simulink model "MT23PED006_SVPWM_OVERMODULATION_SUBHA_DAS"  (R2023b)
settings: Solver=ode23t  StartTime=0.0  StopTime=0.1  MaxStep=1e-6  RelTol=1e-3
model workspace (MAT data in the model file):
  Fs = 2400
  Ma = 0.66
  Ts = 0.000416666666667
  Vdc = 560
  f = 50
libraries: spsVoltageMeasurementLib x6, spsIGBTDiodeLib x6, spsSeriesRLCBranchLib x5, spsGroundLib x2, spsDCVoltageSourceLib x1, dspstat3 x1, spsThreePhaseVIMeasurementLib x1, mcbutilslib x1, sps_lib x1
settings Model: Creator=ixale  LastModifiedBy=ixale
settings DataIOCC: ReturnWorkspaceOutputs=off

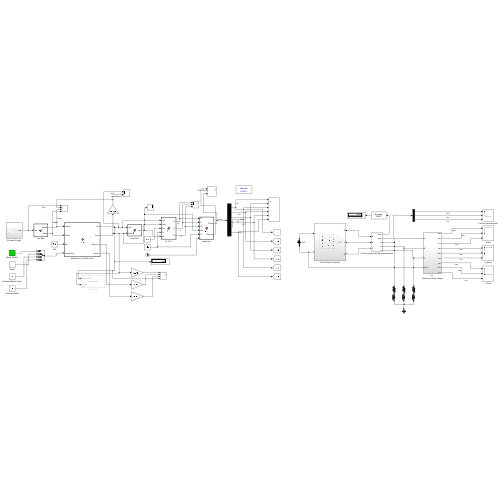
[thumbnail: Simulink's stored preview of the top-level diagram]
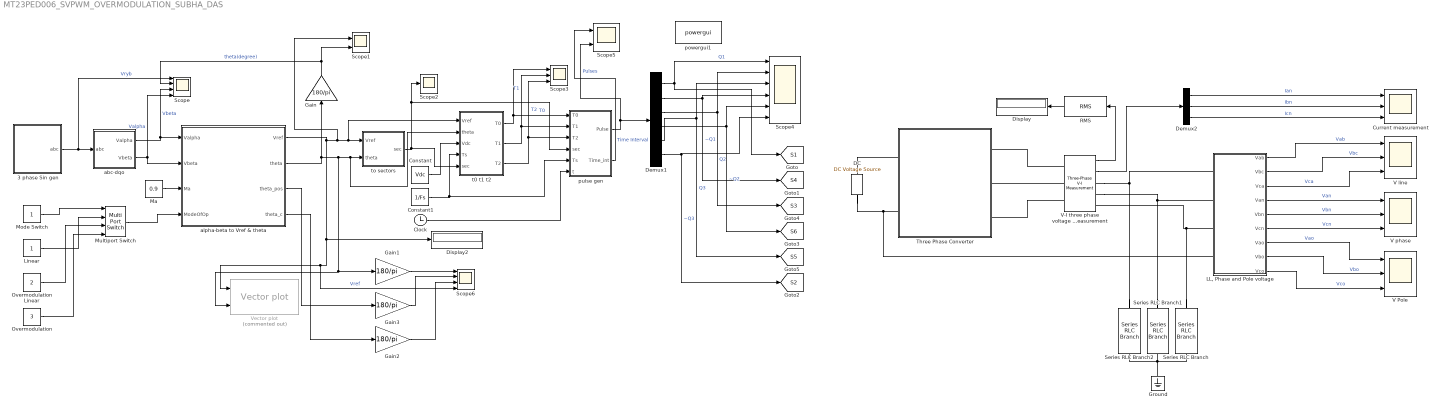
== system MT23PED006_SVPWM_OVERMODULATION_SUBHA_DAS ==
  3 phase Sin gen : Subsystem
  Clock : Clock
      settings: Decimation=100
  Constant : Constant  Value=Vdc
  Constant1 : Constant  Value=1/Fs
  Current measurement : Scope  NumInputPorts=3
  "DC " : spsDCVoltageSourceLib/DC Voltage Source  Amplitude=Vdc  Measurements=None
  Demux1 : Demux  Outputs=6
  Demux2 : Demux  Outputs=3
  Display : Display
  Display2 : Display
  Gain{,1..3} (4 alike) : Gain  Gain=180/pi
  Ground : spsGroundLib/Ground  LConnTagsString=a
  "LL, Phase and Pole voltage" : Subsystem
  Linear : Constant
  Ma : Constant  Value=0.9
  Mode Switch : Constant
  Multiport Switch : MultiPortSwitch  SaturateOnIntegerOverflow=off  InputSameDT=off
  Overmodulation : Constant  Value=3
  Overmodulation Linear : Constant  Value=2
  RMS : dspstat3/RMS  run=on  directionMode=Each column  dimension=1  InputProcessing=Columns as channels (frame based)  reset_popup=None
  Scope : Scope  NumInputPorts=4
  Scope1 : Scope  NumInputPorts=2
  Scope2 : Scope
  Scope3 : Scope  NumInputPorts=3
  Scope4 : Scope  NumInputPorts=6
  Scope5 : Scope  NumInputPorts=2
  Scope6 : Scope  NumInputPorts=4
  Series RLC Branch : spsSeriesRLCBranchLib/Series RLC Branch  LConnTagsString=__new0  RConnTagsString=__new0  BranchType=RL  Resistance=1  Inductance=1e-3  SetiL0=off  InitialCurrent=0  Capacitance=1e-6  Setx0=off  InitialVoltage=0  Measurements=None
  Series RLC Branch1 : spsSeriesRLCBranchLib/Series RLC Branch  LConnTagsString=__new0  RConnTagsString=__new0  BranchType=RL  Resistance=1  Inductance=1e-3  SetiL0=off  InitialCurrent=0  Capacitance=1e-6  Setx0=off  InitialVoltage=0  Measurements=None
  Series RLC Branch2 : spsSeriesRLCBranchLib/Series RLC Branch  LConnTagsString=__new0  RConnTagsString=__new0  BranchType=RL  Resistance=1  Inductance=1e-3  SetiL0=off  InitialCurrent=0  Capacitance=1e-6  Setx0=off  InitialVoltage=0  Measurements=None
  Three Phase Converter : Subsystem
  V Pole : Scope  NumInputPorts=3
  V line : Scope  NumInputPorts=3
  V phase : Scope  NumInputPorts=3
  V-I three phase voltage measurement : spsThreePhaseVIMeasurementLib/Three-Phase V-I Measurement  VoltageMeasurement=phase-to-phase  SetLabelV=off  LabelV=Vabc  Vpu=off  VpuLL=off  CurrentMeasurement=yes  SetLabelI=off  LabelI=Iabc  Ipu=off  Pbase=100e6  Vbase=500e3  OutputType=Complex  PhasorSimulation=off  PSBequivalent=0
  Vector plot : mcbutilslib/Vector plot  Commented=on  InputSignals=Mag Angle  ReferenceFrame=Rotating Reference Frame  axisAlign=D-axis  thetaUnits=Radians  angleUnits=Radians  OpenFigAtSimStart=on  debugEnable=0
      settings: LibrarySourceBlock=mcblib/Signal Management/Vector plot
  abc-dqo : MATLAB Function  TreatAsAtomicUnit=on
  alpha-beta to Vref & theta : MATLAB Function  TreatAsAtomicUnit=on
  powergui1 : sps_lib/powergui  Priority=1  SimulationMode=Discrete  SampleTime=1e-6  frequency=60  Iterations=50  frequencyindice=0  Pbase=100e6  ErrMax=1e-4  UnitsV=kV  UnitsW=MW  buscounter=0  FunctionMessages=off  echomessages=off  EnableUseOfTLC=off  CurrentSourceSwitches=off  DisableSnubberDevices=off  DisableRonSwitches=off  DisableVfSwitches=off  DisplayEquations=off  AutomaticDiscreteSolvers=off  SolverType=Tustin/Backward Euler (TBE)  Interpol=off  ExternalGateDelay=off  methode=off  Ts=100  x0status=blocks  SPID=on  SwTol=0  HookPort=off  NonlinearTolerance=1e-4  nMaxIteration=100  ContinueOnMaxIteration=off  RestoreLinks=warning  ResistiveCurrentMeasurement=off  Frange=[0:2:500]  Ylog=off  Xlog=on  ShowGrid=off  save=off  variable=ZData  structure=0  ZoomFFT=off  StartTime=0.0  cycles=1  DisplayStyle=1  fundamental=60  FreqAxis=off  MaxFrequency=1000  frequencyindicesteady=1  RmsSteady=1  display=off
  pulse gen : MATLAB Function  TreatAsAtomicUnit=on
  t0 t1 t2 : MATLAB Function  TreatAsAtomicUnit=on
  to sectors : MATLAB Function  TreatAsAtomicUnit=on
  tag scope: S1=global, S2=global, S3=global, S4=global, S5=global, S6=global
  wires:
  V-I three phase voltage measurement/1 -> RMS/1
  RMS/1 -> Display/1
  pulse gen/2(Time_int) -> Scope5/1  "Time Interval"
  Demux1/6 -> Scope4/6, [S2]  "~Q3"
  Demux1/5 -> Scope4/3, [S5]  "Q3"
  Demux1/4 -> Scope4/5, [S6]  "~Q2"
  Demux1/3 -> Scope4/2, [S3]  "Q2"
  Demux1/2 -> Scope4/4, [S4]  "~Q1"
  Demux1/1 -> Scope4/1, [S1]  "Q1"
  pulse gen/1(Pulse) -> Scope5/2, Demux1/1  "Pulses"
  Clock/1 -> pulse gen/6(t)
  Gain/1 -> Scope1/2, Scope/2  "theta(degree)"
  t0 t1 t2/1(T0) -> Scope3/1, pulse gen/1(T0)  "T0"
  t0 t1 t2/2(T1) -> Scope3/2, pulse gen/2(T1)  "T1"
  t0 t1 t2/3(T2) -> Scope3/3, pulse gen/3(T2)  "T2"
  Constant1/1 -> pulse gen/5(Ts), t0 t1 t2/4(Ts)
  Constant/1 -> t0 t1 t2/3(Vdc)
  to sectors/1(sec) -> pulse gen/4(sec), Scope2/1, t0 t1 t2/5(sec)
  alpha-beta to Vref & theta/2(theta) -> Gain/1, Gain1/1, Vector plot/2, t0 t1 t2/2(theta), to sectors/2(theta)
  alpha-beta to Vref & theta/1(Vref) -> Scope6/4, Vector plot/1, Display2/1, Scope1/1, t0 t1 t2/1(Vref), to sectors/1(Vref)  "Vref"
  abc-dqo/2(Vbeta) -> Scope/4, alpha-beta to Vref & theta/2(Vbeta)  "Valpha"
  abc-dqo/1(Valpha) -> Scope/3, alpha-beta to Vref & theta/1(Valpha)  "Vbeta"
  3 phase Sin gen/1(abc) -> abc-dqo/1(abc), Scope/1  "Vryb"
  Gain1/1 -> Scope6/1
  Gain2/1 -> Scope6/3
  alpha-beta to Vref & theta/4(theta_c) -> Gain2/1
  alpha-beta to Vref & theta/3(theta_pos) -> Gain3/1
  Gain3/1 -> Scope6/2
  Multiport Switch/1 -> alpha-beta to Vref & theta/4(ModeOfOp)
  Ma/1 -> alpha-beta to Vref & theta/3(Ma)
  Linear/1 -> Multiport Switch/2
  Mode Switch/1 -> Multiport Switch/1
  Overmodulation Linear/1 -> Multiport Switch/3
  Overmodulation/1 -> Multiport Switch/4
  "LL, Phase and Pole voltage"/5(Vbn) -> V phase/2  "Vbn"
  "LL, Phase and Pole voltage"/4(Van) -> V phase/1  "Van"
  "LL, Phase and Pole voltage"/6(Vcn) -> V phase/3  "Vcn"
  "LL, Phase and Pole voltage"/1(Vab) -> V line/1  "Vab"
  "LL, Phase and Pole voltage"/2(Vbc) -> V line/2  "Vbc"
  "LL, Phase and Pole voltage"/3(Vca) -> V line/3  "Vca"
  V-I three phase voltage measurement/2 -> Demux2/1
  Demux2/1 -> Current measurement/1  "Ian"
  Demux2/2 -> Current measurement/2  "Ibn"
  Demux2/3 -> Current measurement/3  "Icn"
  "LL, Phase and Pole voltage"/7(Vao) -> V Pole/1  "Vao"
  "LL, Phase and Pole voltage"/8(Vbo) -> V Pole/2  "Vbo"
  "LL, Phase and Pole voltage"/9(Vco) -> V Pole/3  "Vco"
  connections:
  V-I three phase voltage measurement/RConn2 -- Series RLC Branch1/LConn1 -- "LL, Phase and Pole voltage"/LConn2
  V-I three phase voltage measurement/RConn1 -- Series RLC Branch2/LConn1 -- "LL, Phase and Pole voltage"/LConn1
  Series RLC Branch/LConn1 -- V-I three phase voltage measurement/RConn3 -- "LL, Phase and Pole voltage"/LConn3
  V-I three phase voltage measurement/LConn1 -- Three Phase Converter/RConn1
  Three Phase Converter/LConn1 -- "DC "/RConn1
  V-I three phase voltage measurement/LConn2 -- Three Phase Converter/RConn2
  "DC "/LConn1 -- "LL, Phase and Pole voltage"/LConn4 -- Three Phase Converter/LConn2
  V-I three phase voltage measurement/LConn3 -- Three Phase Converter/RConn3
  Series RLC Branch/RConn1 -- Ground/LConn1 -- Series RLC Branch1/RConn1 -- Series RLC Branch2/RConn1

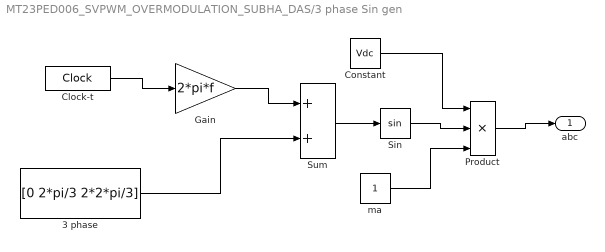
== system MT23PED006_SVPWM_OVERMODULATION_SUBHA_DAS/3 phase Sin gen ==
  3 phase : Constant  Value=[0 2*pi/3 2*2*pi/3]
  Clock-t : DigitalClock  SampleTime=1e-5
  Constant : Constant  Value=Vdc
  Gain : Gain  Gain=2*pi*f
  Product : Product  Inputs=3
  Sin : Trigonometry
  Sum : Sum
  ma : Constant
  abc : Outport
  wires:
  3 phase/1 -> Sum/2
  Gain/1 -> Sum/1
  Clock-t/1 -> Gain/1
  Sum/1 -> Sin/1
  Sin/1 -> Product/2
  Constant/1 -> Product/1
  Product/1 -> abc/1
  ma/1 -> Product/3

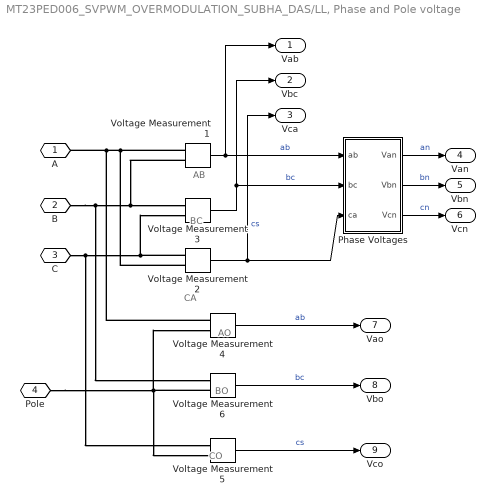
== system MT23PED006_SVPWM_OVERMODULATION_SUBHA_DAS/LL, Phase and Pole voltage ==
  note: CA
  note: BC
  note: AB
  note: CO
  note: BO
  note: AO
  Phase Voltages : MATLAB Function  TreatAsAtomicUnit=on
  Voltage Measurement{1..6} (6 alike) : spsVoltageMeasurementLib/Voltage Measurement  PhasorSimulation=off  OutputType=Complex  PSBequivalent=0
  A : PMIOPort  Side=Left
  B : PMIOPort  Port=2  Side=Left
  C : PMIOPort  Port=3  Side=Left
  Pole : PMIOPort  Port=4  Side=Left
  Vab : Outport
  Vbc : Outport  Port=2
  Vca : Outport  Port=3
  Van : Outport  Port=4
  Vbn : Outport  Port=5
  Vcn : Outport  Port=6
  Vao : Outport  Port=7
  Vbo : Outport  Port=8
  Vco : Outport  Port=9
  wires:
  Voltage Measurement3/1 -> Phase Voltages/2(bc), Vbc/1  "bc"
  Voltage Measurement1/1 -> Phase Voltages/1(ab), Vab/1  "ab"
  Phase Voltages/1(Van) -> Van/1  "an"
  Phase Voltages/2(Vbn) -> Vbn/1  "bn"
  Phase Voltages/3(Vcn) -> Vcn/1  "cn"
  Voltage Measurement2/1 -> Phase Voltages/3(ca), Vca/1  "cs"
  Voltage Measurement4/1 -> Vao/1  "ab"
  Voltage Measurement6/1 -> Vbo/1  "bc"
  Voltage Measurement5/1 -> Vco/1  "cs"
  connections:
  Voltage Measurement1/LConn2 -- Voltage Measurement6/LConn1 -- B/RConn1 -- Voltage Measurement3/LConn1
  Voltage Measurement2/LConn1 -- Voltage Measurement5/LConn1 -- C/RConn1 -- Voltage Measurement3/LConn2
  Voltage Measurement1/LConn1 -- Voltage Measurement4/LConn1 -- A/RConn1 -- Voltage Measurement2/LConn2
  Pole/RConn1 -- Voltage Measurement5/LConn2 -- Voltage Measurement6/LConn2 -- Voltage Measurement4/LConn2

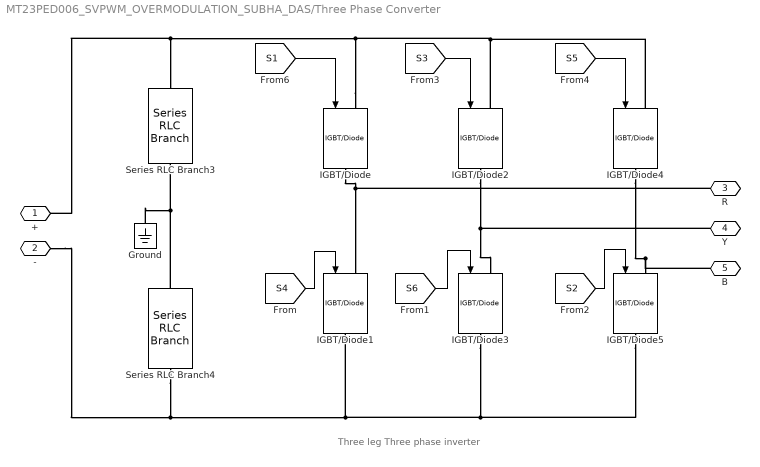
== system MT23PED006_SVPWM_OVERMODULATION_SUBHA_DAS/Three Phase Converter ==
  note: Three leg Three phase inverter
  Ground : spsGroundLib/Ground  LConnTagsString=a
  IGBT/Diode{,1..5} (6 alike) : spsIGBTDiodeLib/IGBT//Diode  Ron=1e-3  Rs=1e5  Cs=inf  Measurements=off
  Series RLC Branch3 : spsSeriesRLCBranchLib/Series RLC Branch  LConnTagsString=__new0  RConnTagsString=__new0  BranchType=RC  Resistance=0.1  Inductance=1e-3  SetiL0=off  InitialCurrent=0  Capacitance=1e-6  Setx0=off  InitialVoltage=0  Measurements=None
  Series RLC Branch4 : spsSeriesRLCBranchLib/Series RLC Branch  LConnTagsString=__new0  RConnTagsString=__new0  BranchType=RC  Resistance=0.1  Inductance=1e-3  SetiL0=off  InitialCurrent=0  Capacitance=1e-6  Setx0=off  InitialVoltage=0  Measurements=None
  + : PMIOPort  Side=Left
  - : PMIOPort  Port=2  Side=Left
  R : PMIOPort  Port=3  Side=Right
  Y : PMIOPort  Port=4  Side=Right
  B : PMIOPort  Port=5  Side=Right
  wires:
  [S6] -> IGBT/Diode3/1
  [S1] -> IGBT/Diode/1
  [S3] -> IGBT/Diode2/1
  [S5] -> IGBT/Diode4/1
  [S4] -> IGBT/Diode1/1
  [S2] -> IGBT/Diode5/1
  connections:
  IGBT/Diode/LConn1 -- Series RLC Branch3/LConn1 -- +/RConn1 -- IGBT/Diode2/LConn1 -- IGBT/Diode4/LConn1
  Series RLC Branch4/LConn1 -- Ground/LConn1 -- Series RLC Branch3/RConn1
  IGBT/Diode5/RConn1 -- IGBT/Diode3/RConn1 -- Series RLC Branch4/RConn1 -- -/RConn1 -- IGBT/Diode1/RConn1
  IGBT/Diode/RConn1 -- R/RConn1 -- IGBT/Diode1/LConn1
  IGBT/Diode5/LConn1 -- B/RConn1 -- IGBT/Diode4/RConn1
  IGBT/Diode2/RConn1 -- Y/RConn1 -- IGBT/Diode3/LConn1

== matlab function MT23PED006_SVPWM_OVERMODULATION_SUBHA_DAS/alpha-beta to Vref & theta ==
  data: Valpha input; Vref output; Vbeta input; Ma input; theta output; theta_pos output; theta_c output; ModeOfOp input
function [Vref, theta, theta_pos, theta_c] = fcn(Valpha, Vbeta, Ma, ModeOfOp)

%z = Valpha + 1i*Vbeta;
%Vref = abs(z);

Vref_c = sqrt(Valpha.^2 + Vbeta.^2); % vref magnitude

%theta = -atan2(imag(z), real(z)); % theta in rad
theta = atan2(Valpha, Vbeta); % theta in rad

% vref modulation

theta_pos = theta;
if theta < 0
    % always take positive value of theta, usually theta goes 0->180 then -180->0.
    % we make it 0->180 then again 0->180
    theta_pos = pi + theta;
end

theta_c = mod(theta_pos,pi/3); % make theta_c 0-59

% make theta_c 0-30 and then 30-0
if theta_c >= pi/6
    theta_c = pi/3 - theta_c;
end

ma = 0.866; % linear region
mode = ModeOfOp;

% linear region
if mode == 1
   %ma = 0.866; % linear region
    ma = Ma;
end

% overmodulation linear
if mode == 2
    ma = 1 -((1-0.866)*(theta_c/(pi/6)));
end

Vref = Vref_c * ma;

== matlab function MT23PED006_SVPWM_OVERMODULATION_SUBHA_DAS/abc-dqo ==
  data: abc input; Valpha output; Vbeta output
function [Valpha, Vbeta] = fcn(abc)

% x = (2*pi*f)* (t - 5e-6); % calculate wt

% getting abc
a = abc(1);
b = abc(2);
c = abc(3);

% matrix for getting alpha beta
T = [1       -1/2        -1/2;...
     0     sqrt(3)/2  -sqrt(3)/2];

U = [a; b; c];

% converting to dq
dq = 2/3 * T * U;

Valpha = dq(1);
Vbeta = dq(2);

== matlab function MT23PED006_SVPWM_OVERMODULATION_SUBHA_DAS/to sectors ==
  data: Vref input; sec output; theta input
function sec  = fcn(Vref, theta)

alpha = 180*theta/pi; % theta in degree
sec = (alpha > 0 & alpha <= 60) * 1 ...
    +(alpha > 60 & alpha <= 120) * 2 ...
    +(alpha > 120 & alpha <= 180) * 3 ...
    +(alpha > -180 & alpha <= -120) * 4 ...
    +(alpha > -120 & alpha <= -60) * 5 ...
    +(alpha > -60 & alpha <= 0) * 6 ...

== matlab function MT23PED006_SVPWM_OVERMODULATION_SUBHA_DAS/t0 t1 t2 ==
  data: Vref input; T0 output; theta input; Vdc input; Ts input; T1 output; T2 output; sec input
function [T0, T1, T2] = fcn(Vref, theta, Vdc, Ts, sec)

theta_dash = theta - (sec - 1) * pi/3;

T1 = Vref/Vdc * Ts * sin(pi/3 - theta_dash)/sin(pi/3);
T2 = Vref/Vdc * Ts * sin(theta_dash)/sin(pi/3);

if (mod(floor(sec),2) ~= 1)  % even sector then swap the timing T0 T1 T2 to T0 T2 T1
    T2 = Vref/Vdc * Ts * sin(pi/3 - theta_dash)/sin(pi/3);
    T1 = Vref/Vdc * Ts * sin(theta_dash)/sin(pi/3);
end

T0 = Ts-T1-T2;

== matlab function MT23PED006_SVPWM_OVERMODULATION_SUBHA_DAS/pulse gen ==
  data: T0 input; Pulse output; T1 input; T2 input; sec input; Ts input; t input; Time_int output
function [Pulse, Time_int]  = fcn(T0, T1, T2, sec, Ts, t)

% sawtooth signal
ref= Ts * rem(t,Ts) / Ts;


% sub interval timings
int1=T0/2;
int2=int1+T1;
int3=int2+T2;
int4=int3+T0/2;
int5=int4+T2;
int6=int5+T1;


Time_int=1+(ref>=int1)+(ref>=int2)+(ref>=int3)+(ref>=int4)+(ref>=int5)+(ref>=int6);

% % format of the array sw_array(x,y,z)
sw_array=zeros(3,7,6);  % initialize the switching table
% % x=[legA Leg B LegC] % y=[Timeint1 timeint2 ..] % Z=[sector1 sector2 ..]
sw_array(:,:,1)=[0	1	1	1	1	1	0;0  0	1	1	1	0	0; 0	0	0	1	0	0	0]; %sector 1
sw_array(:,:,2)=[0	0	1	1	1	0	0;0	 1	1	1	1	1	0; 0	0	0	1	0	0	0]; %sector 2
sw_array(:,:,3)=[0	0	0	1	0	0	0;0	 1	1	1	1	1	0; 0	0	1	1	1	0	0]; %sector 3
sw_array(:,:,4)=[0	0	0	1	0	0	0;0	 0	1	1	1	0	0; 0	1	1	1	1	1	0]; %sector 4
sw_array(:,:,5)=[0	0	1	1	1	0	0;0	 0	0	1	0	0	0; 0	1	1	1	1	1	0]; %sector 5
sw_array(:,:,6)=[0	1	1	1	1	1	0;0	 0	0	1	0	0	0; 0	0	1	1	1	0	0]; %sector 6


% Adding time delay to allow parameter initialization
if t<50e-6
sec=1;
end

S1=sw_array(1,Time_int,sec);
S2= ~S1;
S3=sw_array(2,Time_int,sec);
S4= ~S3;
S5=sw_array(3,Time_int,sec);
S6= ~S5;
% Merged Pulse
Pulse= [S1 S2 S3 S4 S5 S6];


end

== matlab function MT23PED006_SVPWM_OVERMODULATION_SUBHA_DAS/LL, Phase and Pole voltage/Phase Voltages ==
  data: ab input; bc input; ca input; Van output; Vbn output; Vcn output
function [Van, Vbn, Vcn] = voltages(ab, bc, ca)
%VNn= (VaN+VbN+VcN)/3;

% function for phase voltages
Van=(ab-ca)/3;
Vbn=(bc-ab)/3;
Vcn=(ca-bc)/3;
